simulink model "LQR"  (R2025b)
settings: Solver=VariableStepAuto  StartTime=0.0  StopTime=10.0  RelTol=1e-3
undefined symbols (not defined in the file): A, B, K_LQR_i, K_LQR_x, m, n, x0_lmi, xref_lqr
settings Model: Creator=salvo  LastModifiedBy=salvo

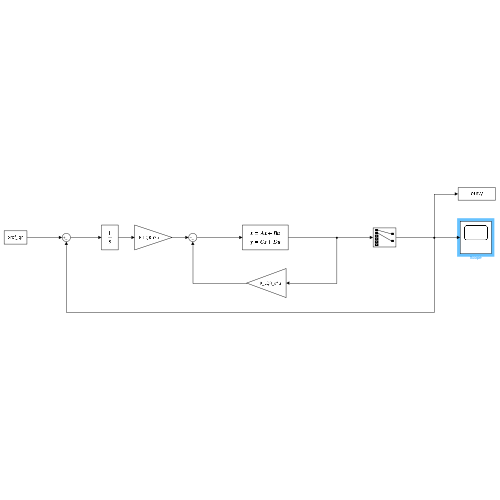
[thumbnail: Simulink's stored preview of the top-level diagram]
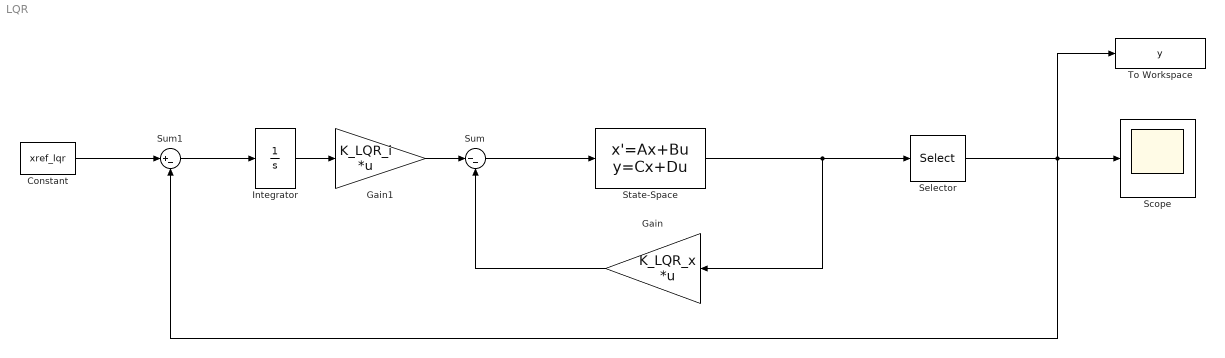
== system LQR ==
  Constant : Constant  Value=xref_lqr
  Gain : Gain  Gain=K_LQR_x  Multiplication=Matrix(K*u)
  Gain1 : Gain  Gain=K_LQR_i  Multiplication=Matrix(K*u)
  Integrator : Integrator
  Scope : Scope
      settings: ActiveDisplayYMinimum=-0.65882775304551788  ActiveDisplayYMaximum=2.5500697426184744
  Selector : Selector  InputPortWidth=6  IndexOptions=Index vector (dialog)  Indices=[1 2]  OutputSizes=1
  State-Space : StateSpace  A=A  B=B  C=eye(n)  D=zeros(n,m)  InitialCondition=x0_lmi
  Sum : Sum  Inputs=|--
  Sum1 : Sum  Inputs=|+-
  To Workspace : ToWorkspace  VariableName=y  SaveFormat=Timeseries  SampleTime=-1
  wires:
  Integrator/1 -> Gain1/1
  Gain1/1 -> Sum/1
  Sum/1 -> State-Space/1
  Gain/1 -> Sum/2
  State-Space/1 -> Gain/1, Selector/1
  Selector/1 -> To Workspace/1, Sum1/2, Scope/1
  Sum1/1 -> Integrator/1
  Constant/1 -> Sum1/1
